simulink model "Ex4_Discrete_Continuous_Sys"  (R2017b)
settings: Solver=VariableStepAuto  StartTime=0.0  StopTime=10.0  RelTol=1e-3
InitFcn:
  | m=0.52;
  | k=155;
  | b=.00144;
undefined symbols (not defined in the file): DiscIntNeverNeededParam
settings Model: Creator=ng8a07e  LastModifiedBy=ng8a07e

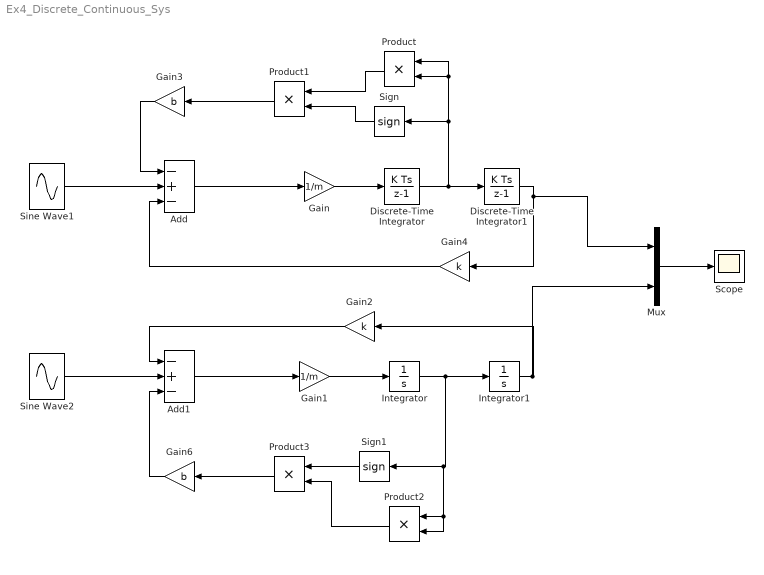
== system Ex4_Discrete_Continuous_Sys ==
  Add : Sum  Inputs=-+-
  Add1 : Sum  Inputs=-+-
  Discrete-Time Integrator : DiscreteIntegrator  InitialConditionSetting=State (most efficient)  SampleTime=-1  ICPrevOutput=DiscIntNeverNeededParam  ICPrevScaledInput=DiscIntNeverNeededParam
  Discrete-Time Integrator1 : DiscreteIntegrator  InitialConditionSetting=State (most efficient)  SampleTime=-1  ICPrevOutput=DiscIntNeverNeededParam  ICPrevScaledInput=DiscIntNeverNeededParam
  Gain : Gain  Gain=1/m
  Gain1 : Gain  Gain=1/m
  Gain2 : Gain  Gain=k
  Gain3 : Gain  Gain=b
  Gain4 : Gain  Gain=k
  Gain6 : Gain  Gain=b
  Integrator : Integrator
  Integrator1 : Integrator
  Mux : Mux  Inputs=2
  Product{,1..3} (4 alike) : Product
  Scope : Scope
  Sign : Signum
  Sign1 : Signum
  Sine Wave1 : Sin  Amplitude=2.3  Frequency=131  SampleTime=0.01
  Sine Wave2 : Sin  Amplitude=2.3  Frequency=131  SampleTime=0
  wires:
  Sine Wave1/1 -> Add/2
  Sine Wave2/1 -> Add1/2
  Gain3/1 -> Add/1
  Gain6/1 -> Add1/3
  Add1/1 -> Gain1/1
  Add/1 -> Gain/1
  Gain/1 -> Discrete-Time Integrator/1
  Discrete-Time Integrator/1 -> Product/2, Product/1, Sign/1, Discrete-Time Integrator1/1
  Gain1/1 -> Integrator/1
  Integrator/1 -> Product2/2, Product2/1, Sign1/1, Integrator1/1
  Product3/1 -> Gain6/1
  Sign1/1 -> Product3/1
  Product2/1 -> Product3/2
  Sign/1 -> Product1/2
  Product/1 -> Product1/1
  Product1/1 -> Gain3/1
  Integrator1/1 -> Mux/2, Gain2/1
  Discrete-Time Integrator1/1 -> Mux/1, Gain4/1
  Gain4/1 -> Add/3
  Gain2/1 -> Add1/1
  Mux/1 -> Scope/1
